simulink model "pwm_deadtime_sampling_model"  (R2023b)
settings: Solver=FixedStepDiscrete  StartTime=0.0  StopTime=pwm_sampling_defaults.simcfg.stop_time  FixedStep=pwm_sampling_defaults.simcfg.Ts_step  RelTol=1e-3
values from neighbouring files (symbols this model uses):
  AdcSettleTime_s = 9.9999999747524271E-7    [pwm_deadtime_sampling_interface.sldd]
  DeadTimeTotal_s = 9.9999999747524271E-7    [pwm_deadtime_sampling_interface.sldd]
  MinValidWindow_s = 2.4999999368446879E-6    [pwm_deadtime_sampling_interface.sldd]
  PwmPeriod_s = 4.9999998736893758E-5    [pwm_deadtime_sampling_interface.sldd]
undefined symbols (not defined in the file or in its folder): pwm_sampling_defaults, pwm_sampling_test
settings Model: DataDictionary=pwm_deadtime_sampling_interface.sldd  Creator=user  LastModifiedBy=user
settings OptimizationCC: DefaultParameterBehavior=Inlined  EnhancedBackFolding=on  PassReuseOutputArgsAs=Individual arguments  OptimizeBlockOrder=speed  DifferentSizesBufferReuse=on  OptimizationCustomize=off  EfficientTunableParamExpr=on
settings DebuggingCC: ParameterTunabilityLossMsg=error
settings HardwareCC: ProdBitPerPointer=32  ProdBitPerSizeT=32  ProdBitPerPtrDiffT=32  ProdLargestAtomicInteger=Long  ProdLargestAtomicFloat=Double  ProdWordSize=32  ProdHWDeviceType=ARM Compatible->ARM Cortex  TargetLargestAtomicInteger=Long  TargetLargestAtomicFloat=Double  TargetIntDivRoundTo=Zero  TargetEndianess=LittleEndian  TargetHWDeviceType=ARM Compatible->ARM Cortex  ProdEqTarget=off
settings SFSimCC: MATLABDynamicMemAlloc=off
settings RTWCC: Description=Embedded Coder  SystemTargetFile=ert.tlc  GenCodeOnly=on  TemplateMakefile=ert_default_tmf  GenerateReport=on
settings CodeAppCC: ForceParamTrailComments=on  IgnoreCustomStorageClasses=off  OperatorAnnotations=on  SimulinkDataObjDesc=on  SFDataObjDesc=on  InsertBlockDesc=on
settings ERTTargetCC: TargetLangStandard=C99 (ISO)  CodeInterfacePackaging=Reusable function  InlinedParameterPlacement=NonHierarchical  ERTCustomFileTemplate=example_file_process.tlc

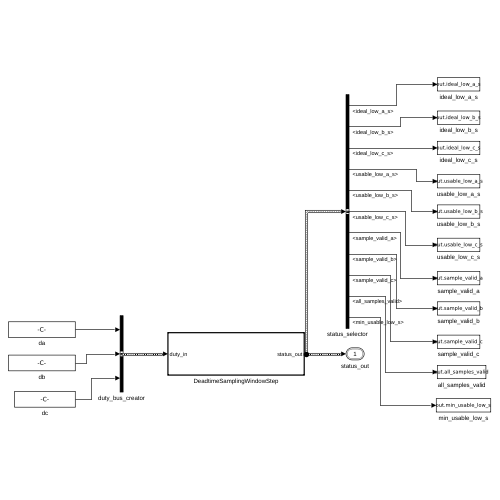
[thumbnail: Simulink's stored preview of the top-level diagram]
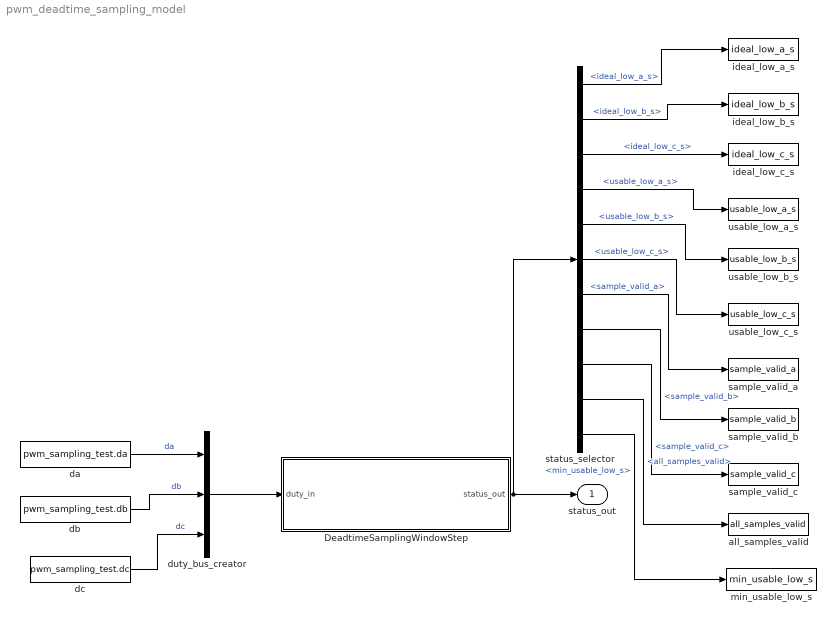
== system pwm_deadtime_sampling_model ==
  DeadtimeSamplingWindowStep : Subsystem  TreatAsAtomicUnit=on  RTWFcnName=DeadtimeSamplingWindowStep  RTWFileName=DeadtimeSamplingWindowStep
      settings: RTWFcnNameOpts=User specified  RTWFileNameOpts=User specified
  all_samples_valid : ToWorkspace  VariableName=all_samples_valid  SaveFormat=Structure With Time  SampleTime=-1
  da : Constant  Value=pwm_sampling_test.da  OutDataTypeStr=T_PwmDuty  SampleTime=pwm_sampling_defaults.simcfg.Ts_step
  db : Constant  Value=pwm_sampling_test.db  OutDataTypeStr=T_PwmDuty  SampleTime=pwm_sampling_defaults.simcfg.Ts_step
  dc : Constant  Value=pwm_sampling_test.dc  OutDataTypeStr=T_PwmDuty  SampleTime=pwm_sampling_defaults.simcfg.Ts_step
  duty_bus_creator : BusCreator  Inputs=3  OutDataTypeStr=Bus: pwm_phase_duty_t  NonVirtualBus=on
  ideal_low_a_s : ToWorkspace  VariableName=ideal_low_a_s  SaveFormat=Structure With Time  SampleTime=-1
  ideal_low_b_s : ToWorkspace  VariableName=ideal_low_b_s  SaveFormat=Structure With Time  SampleTime=-1
  ideal_low_c_s : ToWorkspace  VariableName=ideal_low_c_s  SaveFormat=Structure With Time  SampleTime=-1
  min_usable_low_s : ToWorkspace  VariableName=min_usable_low_s  SaveFormat=Structure With Time  SampleTime=-1
  sample_valid_a : ToWorkspace  VariableName=sample_valid_a  SaveFormat=Structure With Time  SampleTime=-1
  sample_valid_b : ToWorkspace  VariableName=sample_valid_b  SaveFormat=Structure With Time  SampleTime=-1
  sample_valid_c : ToWorkspace  VariableName=sample_valid_c  SaveFormat=Structure With Time  SampleTime=-1
  status_selector : BusSelector  OutputSignals=ideal_low_a_s,ideal_low_b_s,ideal_low_c_s,usable_low_a_s,usable_low_b_s,usable_low_c_s,sample_valid_a,sample_valid_b,sample_valid_c,all_samples_valid,min_usable_low_s
  usable_low_a_s : ToWorkspace  VariableName=usable_low_a_s  SaveFormat=Structure With Time  SampleTime=-1
  usable_low_b_s : ToWorkspace  VariableName=usable_low_b_s  SaveFormat=Structure With Time  SampleTime=-1
  usable_low_c_s : ToWorkspace  VariableName=usable_low_c_s  SaveFormat=Structure With Time  SampleTime=-1
  status_out : Outport  OutDataTypeStr=Bus: pwm_sampling_status_t  PortDimensions=1
  wires:
  status_selector/11 -> min_usable_low_s/1  "<min_usable_low_s>"
  status_selector/10 -> all_samples_valid/1  "<all_samples_valid>"
  dc/1 -> duty_bus_creator/3  "dc"
  duty_bus_creator/1 -> DeadtimeSamplingWindowStep/1(duty_in)
  db/1 -> duty_bus_creator/2  "db"
  DeadtimeSamplingWindowStep/1(status_out) -> status_selector/1, status_out/1
  da/1 -> duty_bus_creator/1  "da"
  status_selector/7 -> sample_valid_a/1  "<sample_valid_a>"
  status_selector/9 -> sample_valid_c/1  "<sample_valid_c>"
  status_selector/1 -> ideal_low_a_s/1  "<ideal_low_a_s>"
  status_selector/2 -> ideal_low_b_s/1  "<ideal_low_b_s>"
  status_selector/3 -> ideal_low_c_s/1  "<ideal_low_c_s>"
  status_selector/4 -> usable_low_a_s/1  "<usable_low_a_s>"
  status_selector/5 -> usable_low_b_s/1  "<usable_low_b_s>"
  status_selector/6 -> usable_low_c_s/1  "<usable_low_c_s>"
  status_selector/8 -> sample_valid_b/1  "<sample_valid_b>"

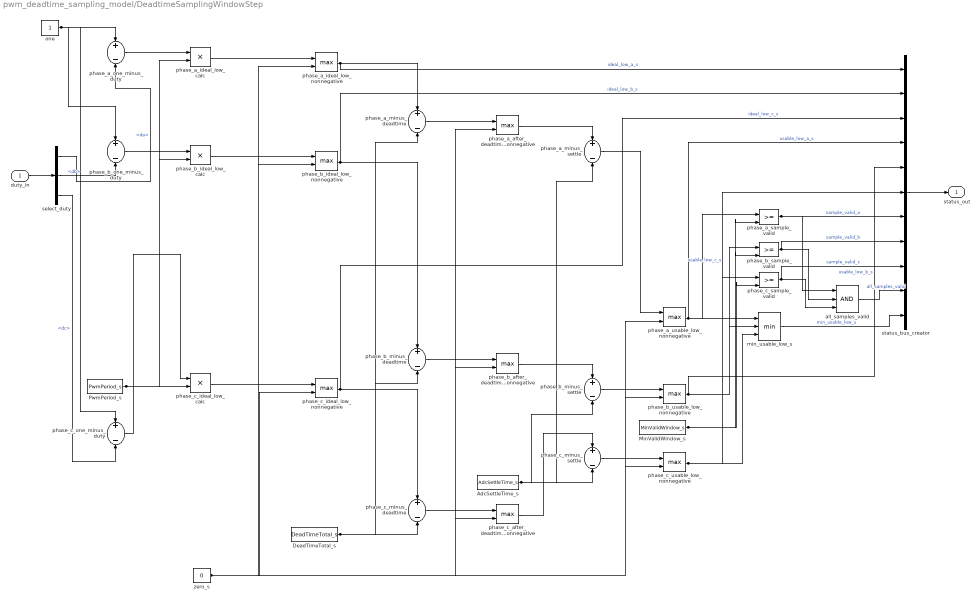
== system pwm_deadtime_sampling_model/DeadtimeSamplingWindowStep ==
  duty_in : Inport  OutDataTypeStr=Bus: pwm_phase_duty_t  PortDimensions=1  BusOutputAsStruct=on
  AdcSettleTime_s : Constant  Value=AdcSettleTime_s  OutDataTypeStr=T_PwmTime  SampleTime=-1
  DeadTimeTotal_s : Constant  Value=DeadTimeTotal_s  OutDataTypeStr=T_PwmTime  SampleTime=-1
  MinValidWindow_s : Constant  Value=MinValidWindow_s  OutDataTypeStr=T_PwmTime  SampleTime=-1
  PwmPeriod_s : Constant  Value=PwmPeriod_s  OutDataTypeStr=T_PwmTime  SampleTime=-1
  all_samples_valid : Logic  Inputs=3  AllPortsSameDT=off  OutDataTypeStr=T_PwmSampleValid
  min_usable_low_s : MinMax  Inputs=3  OutDataTypeStr=T_PwmTime
  one : Constant  OutDataTypeStr=T_PwmSamplingFloat  SampleTime=-1
  phase_a_after_deadtime_nonnegative : MinMax  Function=max  Inputs=2  OutDataTypeStr=T_PwmTime
  phase_a_ideal_low_calc : Product  Inputs=**  OutDataTypeStr=T_PwmTime
  phase_a_ideal_low_nonnegative : MinMax  Function=max  Inputs=2  OutDataTypeStr=T_PwmTime
  phase_a_minus_deadtime : Sum  Inputs=+-  OutDataTypeStr=T_PwmTime
  phase_a_minus_settle : Sum  Inputs=+-  OutDataTypeStr=T_PwmTime
  phase_a_one_minus_duty : Sum  Inputs=+-  OutDataTypeStr=T_PwmSamplingFloat
  phase_a_sample_valid : RelationalOperator  OutDataTypeStr=boolean  RndMeth=Simplest  InputSameDT=off
  phase_a_usable_low_nonnegative : MinMax  Function=max  Inputs=2  OutDataTypeStr=T_PwmTime
  phase_b_after_deadtime_nonnegative : MinMax  Function=max  Inputs=2  OutDataTypeStr=T_PwmTime
  phase_b_ideal_low_calc : Product  Inputs=**  OutDataTypeStr=T_PwmTime
  phase_b_ideal_low_nonnegative : MinMax  Function=max  Inputs=2  OutDataTypeStr=T_PwmTime
  phase_b_minus_deadtime : Sum  Inputs=+-  OutDataTypeStr=T_PwmTime
  phase_b_minus_settle : Sum  Inputs=+-  OutDataTypeStr=T_PwmTime
  phase_b_one_minus_duty : Sum  Inputs=+-  OutDataTypeStr=T_PwmSamplingFloat
  phase_b_sample_valid : RelationalOperator  OutDataTypeStr=boolean  RndMeth=Simplest  InputSameDT=off
  phase_b_usable_low_nonnegative : MinMax  Function=max  Inputs=2  OutDataTypeStr=T_PwmTime
  phase_c_after_deadtime_nonnegative : MinMax  Function=max  Inputs=2  OutDataTypeStr=T_PwmTime
  phase_c_ideal_low_calc : Product  Inputs=**  OutDataTypeStr=T_PwmTime
  phase_c_ideal_low_nonnegative : MinMax  Function=max  Inputs=2  OutDataTypeStr=T_PwmTime
  phase_c_minus_deadtime : Sum  Inputs=+-  OutDataTypeStr=T_PwmTime
  phase_c_minus_settle : Sum  Inputs=+-  OutDataTypeStr=T_PwmTime
  phase_c_one_minus_duty : Sum  Inputs=+-  OutDataTypeStr=T_PwmSamplingFloat
  phase_c_sample_valid : RelationalOperator  OutDataTypeStr=boolean  RndMeth=Simplest  InputSameDT=off
  phase_c_usable_low_nonnegative : MinMax  Function=max  Inputs=2  OutDataTypeStr=T_PwmTime
  select_duty : BusSelector  OutputSignals=da,db,dc
  status_bus_creator : BusCreator  Inputs=11  OutDataTypeStr=Bus: pwm_sampling_status_t  NonVirtualBus=on
  zero_s : Constant  Value=0  OutDataTypeStr=T_PwmTime  SampleTime=-1
  status_out : Outport  OutDataTypeStr=Bus: pwm_sampling_status_t  PortDimensions=1
  wires:
  status_bus_creator/1 -> status_out/1
  all_samples_valid/1 -> status_bus_creator/10  "all_samples_valid"
  phase_c_sample_valid/1 -> all_samples_valid/3, status_bus_creator/9  "sample_valid_c"
  phase_c_usable_low_nonnegative/1 -> min_usable_low_s/3, status_bus_creator/6, phase_c_sample_valid/1  "usable_low_c_s"
  MinValidWindow_s/1 -> phase_b_sample_valid/2, phase_c_sample_valid/2, phase_a_sample_valid/2
  zero_s/1 -> phase_c_ideal_low_nonnegative/2, phase_b_ideal_low_nonnegative/2, phase_a_ideal_low_nonnegative/2, phase_b_usable_low_nonnegative/2, phase_a_usable_low_nonnegative/2, phase_c_usable_low_nonnegative/2, phase_a_after_deadtime_nonnegative/2, phase_c_after_deadtime_nonnegative/2, phase_b_after_deadtime_nonnegative/2
  phase_c_ideal_low_calc/1 -> phase_c_ideal_low_nonnegative/1
  phase_a_ideal_low_calc/1 -> phase_a_ideal_low_nonnegative/1
  phase_b_one_minus_duty/1 -> phase_b_ideal_low_calc/1
  phase_b_after_deadtime_nonnegative/1 -> phase_b_minus_settle/1
  min_usable_low_s/1 -> status_bus_creator/11  "min_usable_low_s"
  phase_a_sample_valid/1 -> all_samples_valid/1, status_bus_creator/7  "sample_valid_a"
  PwmPeriod_s/1 -> phase_b_ideal_low_calc/2, phase_c_ideal_low_calc/2, phase_a_ideal_low_calc/2
  phase_c_minus_settle/1 -> phase_c_usable_low_nonnegative/1
  phase_b_usable_low_nonnegative/1 -> min_usable_low_s/2, phase_b_sample_valid/1, status_bus_creator/5  "usable_low_b_s"
  phase_a_one_minus_duty/1 -> phase_a_ideal_low_calc/1
  select_duty/3 -> phase_c_one_minus_duty/2  "<dc>"
  phase_a_usable_low_nonnegative/1 -> min_usable_low_s/1, phase_a_sample_valid/1, status_bus_creator/4  "usable_low_a_s"
  one/1 -> phase_b_one_minus_duty/1, phase_a_one_minus_duty/1, phase_c_one_minus_duty/1
  phase_c_one_minus_duty/1 -> phase_c_ideal_low_calc/1
  duty_in/1 -> select_duty/1
  phase_a_ideal_low_nonnegative/1 -> status_bus_creator/1, phase_a_minus_deadtime/1  "ideal_low_a_s"
  phase_b_sample_valid/1 -> all_samples_valid/2, status_bus_creator/8  "sample_valid_b"
  phase_c_ideal_low_nonnegative/1 -> status_bus_creator/3, phase_c_minus_deadtime/1  "ideal_low_c_s"
  phase_b_ideal_low_nonnegative/1 -> status_bus_creator/2, phase_b_minus_deadtime/1  "ideal_low_b_s"
  select_duty/1 -> phase_a_one_minus_duty/2  "<da>"
  DeadTimeTotal_s/1 -> phase_a_minus_deadtime/2, phase_c_minus_deadtime/2, phase_b_minus_deadtime/2
  phase_a_minus_deadtime/1 -> phase_a_after_deadtime_nonnegative/1
  phase_b_minus_deadtime/1 -> phase_b_after_deadtime_nonnegative/1
  phase_c_minus_deadtime/1 -> phase_c_after_deadtime_nonnegative/1
  phase_a_after_deadtime_nonnegative/1 -> phase_a_minus_settle/1
  AdcSettleTime_s/1 -> phase_a_minus_settle/2, phase_b_minus_settle/2, phase_c_minus_settle/2
  phase_c_after_deadtime_nonnegative/1 -> phase_c_minus_settle/1
  select_duty/2 -> phase_b_one_minus_duty/2  "<db>"
  phase_a_minus_settle/1 -> phase_a_usable_low_nonnegative/1
  phase_b_ideal_low_calc/1 -> phase_b_ideal_low_nonnegative/1
  phase_b_minus_settle/1 -> phase_b_usable_low_nonnegative/1
